simulink model "Modelo_SIR"  (R2021b)
settings: Solver=VariableStepAuto  StartTime=0.0  StopTime=100.0  RelTol=1e-3
undefined symbols (not defined in the file): beta, I0, r, R0, S0
settings Model: Creator=19.00610-0  LastModifiedBy=19.00610-0

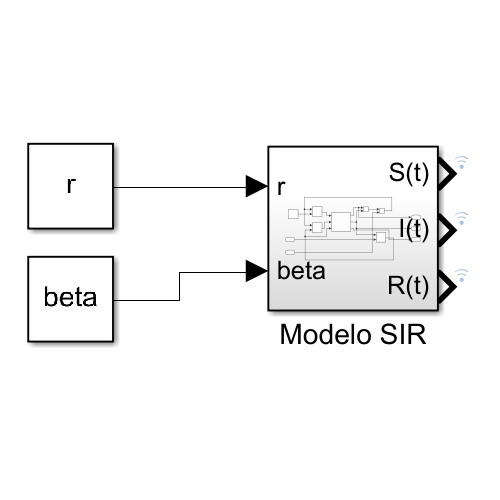
[thumbnail: Simulink's stored preview of the top-level diagram]
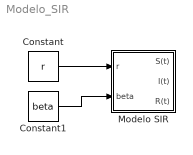
== system Modelo_SIR ==
  Constant : Constant  Value=r
  Constant1 : Constant  Value=beta
  Modelo SIR : Subsystem
  wires:
  Constant/1 -> Modelo SIR/1(r)
  Constant1/1 -> Modelo SIR/2(beta)

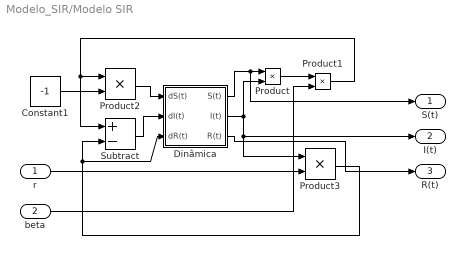
== system Modelo_SIR/Modelo SIR ==
  r : Inport
  beta : Inport  Port=2
  Constant1 : Constant  Value=-1
  Dinâmica : Subsystem
  Product{,1..3} (4 alike) : Product
  Subtract : Sum  Inputs=+-
  S(t) : Outport
  I(t) : Outport  Port=2
  R(t) : Outport  Port=3
  wires:
  Dinâmica/2(I(t)) -> I(t)/1, Product3/1, Product/2
  Dinâmica/1(S(t)) -> S(t)/1, Product/1
  Product2/1 -> Dinâmica/1(dS(t))
  Product1/1 -> Product2/1, Subtract/1
  Product3/1 -> Dinâmica/3(dR(t)), Subtract/2
  Dinâmica/3(R(t)) -> R(t)/1
  Product/1 -> Product1/1
  Subtract/1 -> Dinâmica/2(dI(t))
  Constant1/1 -> Product2/2
  beta/1 -> Product1/2
  r/1 -> Product3/2

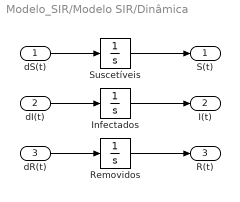
== system Modelo_SIR/Modelo SIR/Dinâmica ==
  dS(t) : Inport
  dI(t) : Inport  Port=2
  dR(t) : Inport  Port=3
  Infectados : Integrator  InitialCondition=I0
  Removidos : Integrator  InitialCondition=R0
  Suscetíveis : Integrator  InitialCondition=S0
  S(t) : Outport
  I(t) : Outport  Port=2
  R(t) : Outport  Port=3
  wires:
  Infectados/1 -> I(t)/1
  dR(t)/1 -> Removidos/1
  Removidos/1 -> R(t)/1
  Suscetíveis/1 -> S(t)/1
  dI(t)/1 -> Infectados/1
  dS(t)/1 -> Suscetíveis/1
